simulink model "ex8impsliding2"  (R2025b)
settings: Solver=ode4  StartTime=0.0  StopTime=10.0  FixedStep=0.05  RelTol=1e-3
settings Model: Creator=Esteban  LastModifiedBy=Esteban

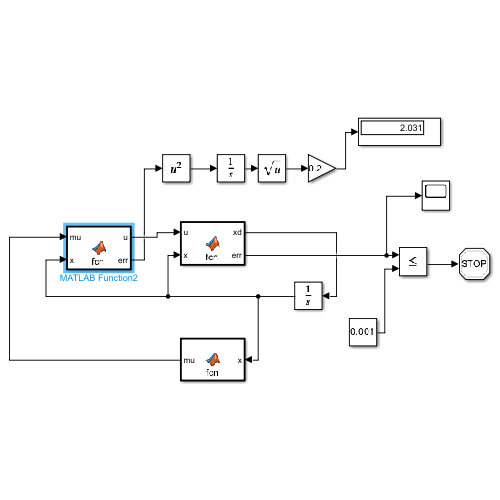
[thumbnail: Simulink's stored preview of the top-level diagram]
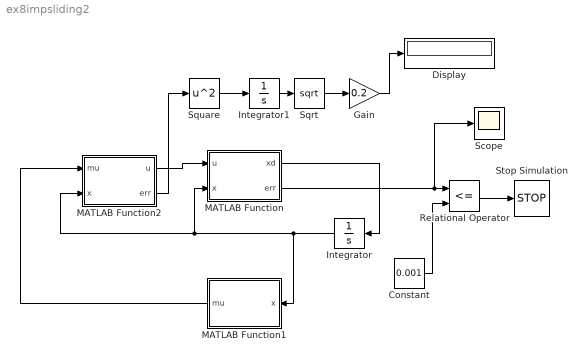
== system ex8impsliding2 ==
  Constant : Constant  Value=0.001
  Display : Display
  Gain : Gain  Gain=0.2
  Integrator : Integrator  InitialCondition=[-7/2;4]
  Integrator1 : Integrator
  MATLAB Function : MATLAB Function  TreatAsAtomicUnit=on
  MATLAB Function1 : MATLAB Function  TreatAsAtomicUnit=on
  MATLAB Function2 : MATLAB Function  TreatAsAtomicUnit=on
  Relational Operator : RelationalOperator  Operator=<=  OutDataTypeStr=boolean  RndMeth=Simplest  InputSameDT=off
  Scope : Scope
      settings: ActiveDisplayYMinimum=-0.436485155229997  ActiveDisplayYMaximum=3.9373872394699996
  Sqrt : Sqrt
  Square : Math  Operator=square
  Stop Simulation : Stop
  wires:
  MATLAB Function/1(xd) -> Integrator/1
  Integrator/1 -> MATLAB Function1/1(x), MATLAB Function/2(x), MATLAB Function2/2(x)
  MATLAB Function1/1(mu) -> MATLAB Function2/1(mu)
  MATLAB Function2/1(u) -> MATLAB Function/1(u)
  Constant/1 -> Relational Operator/2
  MATLAB Function/2(err) -> Scope/1, Relational Operator/1
  Relational Operator/1 -> Stop Simulation/1
  MATLAB Function2/2(err) -> Square/1
  Square/1 -> Integrator1/1
  Integrator1/1 -> Sqrt/1
  Sqrt/1 -> Gain/1
  Gain/1 -> Display/1

== matlab function ex8impsliding2/MATLAB Function ==
  data: xd output; u input; err output; x input
function [xd,err] = fcn(u,x)

xd = [x(2);
    0.2*x(1)^3+x(1)-u-3*x(2)];

y = x(1);

err = norm(y);

== matlab function ex8impsliding2/MATLAB Function2 ==
  data: mu input; u output; x input; err output
function [u,err] = fcn(mu,x)

k1 = 5;
k2 = 12;
n = 1;
s = mu(2) + k2*mu(1);

v = - k2*mu(2) - k1*tanh(s*n);

u = x(1)^3/5 + x(1) - v - 3*x(2);

err = norm(u);

== matlab function ex8impsliding2/MATLAB Function1 ==
  data: x input; mu output
function mu = fcn(x)

mu = [x(1);x(2)];
